simulink model "integraYdisparaSIM"  (Simulink 7.5)
settings: Solver=ode3  StartTime=0.0  StopTime=20.0  FixedStep=0.001  MaxStep=.02  MinStep=.02  RelTol=1e-3
values from neighbouring files (symbols this model uses):
  C = 100e-6    (= 0.0001)    [integraYdispara.m]
  R = 47e3    (= 47000)    [integraYdispara.m]
  Ubat = 5    [integraYdispara.m]
libraries: simulink x1
settings Model: Creator=Mariano  LastModifiedBy=Mariano
settings SolverCC: InitialStep=0.02

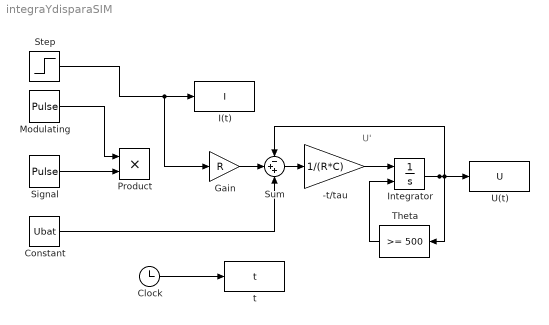
== system integraYdisparaSIM ==
  note: U'
  -t/tau : Gain  Gain=1/(R*C)  ParameterDataType=fixdt(1, 16)  ParameterScaling=2^0  OutDataType=fixdt(1, 16)  OutScaling=2^0
  Clock : Clock
      settings: Decimation=10
  Constant : Constant  Value=Ubat  OutDataType=fixdt(1, 16)  OutScaling=2^0
  Gain : Gain  Gain=R  ParameterDataType=fixdt(1, 16)  ParameterScaling=2^0  OutDataType=fixdt(1, 16)  OutScaling=2^0
  I(t) : ToWorkspace  VariableName=I  SampleTime=-1  SaveFormat=Array
  Integrator : Integrator  ExternalReset=rising  InitialCondition=Ubat
  Modulating : DiscretePulseGenerator  PulseType=Time based  Amplitude=0.1  Period=1  PulseWidth=.5  PhaseDelay=1  SampleTime=1
  Product : Product  OutDataType=fixdt(1, 16)  OutScaling=2^0  RndMeth=Zero
  Signal : DiscretePulseGenerator  PulseType=Time based  Amplitude=1  Period=21  PulseWidth=25  PhaseDelay=0  SampleTime=1
  Step : Step  After=.100  SampleTime=0
  Sum : Sum  Inputs=-++  OutDataType=fixdt(1, 16)  OutScaling=2^0
  Theta : simulink/Logic and Bit Operations/Compare To Constant  SystemSampleTime=-1  relop=>=  const=500  LogicOutDataTypeMode=boolean
  U(t) : ToWorkspace  VariableName=U  SampleTime=-1  SaveFormat=Array
  t : ToWorkspace  VariableName=t  SampleTime=-1  SaveFormat=Array
  wires:
  Integrator/1 -> Sum/1, U(t)/1, Theta/1
  -t/tau/1 -> Integrator/1
  Sum/1 -> -t/tau/1
  Gain/1 -> Sum/2
  Constant/1 -> Sum/3
  Signal/1 -> Product/2
  Modulating/1 -> Product/1
  Clock/1 -> t/1
  Theta/1 -> Integrator/2
  Step/1 -> I(t)/1, Gain/1
